simulink model "p2"  (R2020a)
settings: Solver=VariableStepAuto  StartTime=0.0  StopTime=5000  RelTol=1e-3
settings Model: Creator=007  LastModifiedBy=007

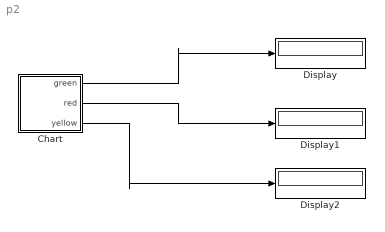
== system p2 ==
  Chart : Stateflow chart  TreatAsAtomicUnit=on
  Display : Display
  Display1 : Display
  Display2 : Display
  wires:
  Chart/1(green) -> Display/1
  Chart/2(red) -> Display1/1
  Chart/3(yellow) -> Display2/1

== stateflow chart p2/Chart ==
  state Go
    entry:
    red=0;
    yellow=0;
    green=1;
  state PrepareToStop
    entry:
    red=0;
    yellow=1;
    green=0;
  state Stop
    entry:
    red=1;
    yellow=0;
    green=0;
  (default) -> Stop
  PrepareToStop -> Go : after(10,sec)
  Stop -> PrepareToStop : after(10,sec)
  Go -> Stop : after(30,sec)
  data: green output; red output; yellow output
